simulink model "h"  (R2024a)
settings: Solver=ode45  StartTime=0.0  StopTime=1.5  RelTol=1e-3
PreLoadFcn:
  | power_PVarray_250kW_param;
InitFcn:
  | power_PVarray_250kW_param;
undefined symbols (not defined in the file or in its folder): Clink, D1, Delta, Fc, Fnom, Increment_MPPT, k1, k2, Ki_Ireg, Ki_VDCreg, Kp_Ireg, Kp_VDCreg, LimitL_Ireg, Limits_MPPT, LimitU_Ireg, Pnom, Pnom_xfo, RL, RLff, sigbuilder_block, Ts_Control, Ts_Power, Vf, Vfd, Vnom_dc, Vnom_prim, Vnom_sec
libraries: spsThreePhaseParallelRLCLoadLib x3, spsSeriesRLCBranchLib x3, spsThreePhaseTransformerTwoWindingsLib x2, spsDistributedParametersLineLib x2, eeGeneralControl x2, slpidlib x2, spsabctodq0Lib x2, spsMeanLib x2, spsVoltageMeasurementLib x2, spsThreePhaseSourceLib x1, spsThreeLevelBridgeLib x1, spsThreePhaseVIMeasurementLib x1
Description:
  | Copyright 2008-2018 The MathWorks, Inc.
settings Model: Creator=MathWorks  LastModifiedBy=Ahmed
settings SolverCC: AlgebraicLoopSolver=TrustRegion
settings DataIOCC: LimitDataPoints=on  SaveFormat=Array  SignalLoggingSaveFormat=ModelDataLogs  SignalLogging=off  DSMLogging=off  ReturnWorkspaceOutputs=off
settings OptimizationCC: ExpressionDepthLimit=2147483647  LifeSpan=inf
settings DebuggingCC: UnderspecifiedInitializationDetection=Classic  MergeDetectMultiDrivingBlocksExec=none  SolverPrmCheckMsg=warning  FcnCallInpInsideContextMsg=warning  UnconnectedInputMsg=warning  UnconnectedOutputMsg=warning  UnconnectedLineMsg=warning  StateNameClashWarn=warning  SFUnexpectedBacktrackingDiag=warning  SFNoUnconditionalDefaultTransitionDiag=warning  SFExecutionAtInitializationDiag=none  ArithmeticOperatorsInVariantConditions=warning
settings HardwareCC: ProdBitPerPointer=32  ProdBitPerSizeT=32  ProdBitPerPtrDiffT=32  ProdLargestAtomicFloat=None  ProdIntDivRoundTo=Undefined  ProdEndianess=Unspecified  ProdWordSize=32  ProdHWDeviceType=32-bit Generic
settings ModelReferenceCC: EnableRefExpFcnMdlSchedulingChecks=on  PropagateSignalLabelsOutOfModel=off
settings SFSimCC: SimUseLocalCustomCode=off  CustomCodeUndefinedFunction=UseInterfaceOnly
settings RTWCC: RTWUseLocalCustomCode=off  GPUComputeCapability=3.5
settings CodeAppCC: StateflowObjectComments=on
settings GRTTargetCC: TargetLangStandard=C89/C90 (ANSI)  CombineOutputUpdateFcns=off  GRTInterface=on
settings ConfigComp: CovMetricSettings=dw  CovSaveCumulativeToWorkspaceVar=on  CovSaveSingleToWorkspaceVar=on  CovExternalEMLEnable=off  CovSFcnEnable=off
settings SimscapeCC: SimscapeNormalizeSystem=off

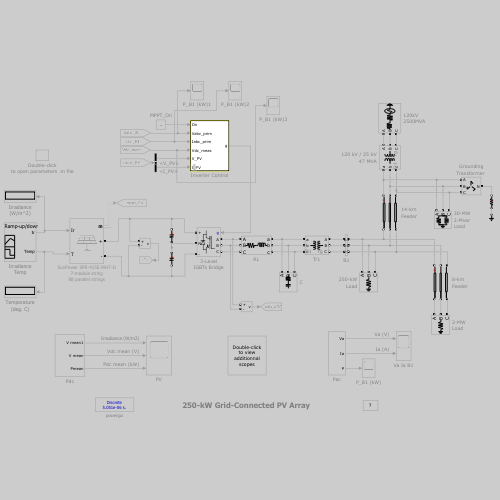
[thumbnail: Simulink's stored preview of the top-level diagram]
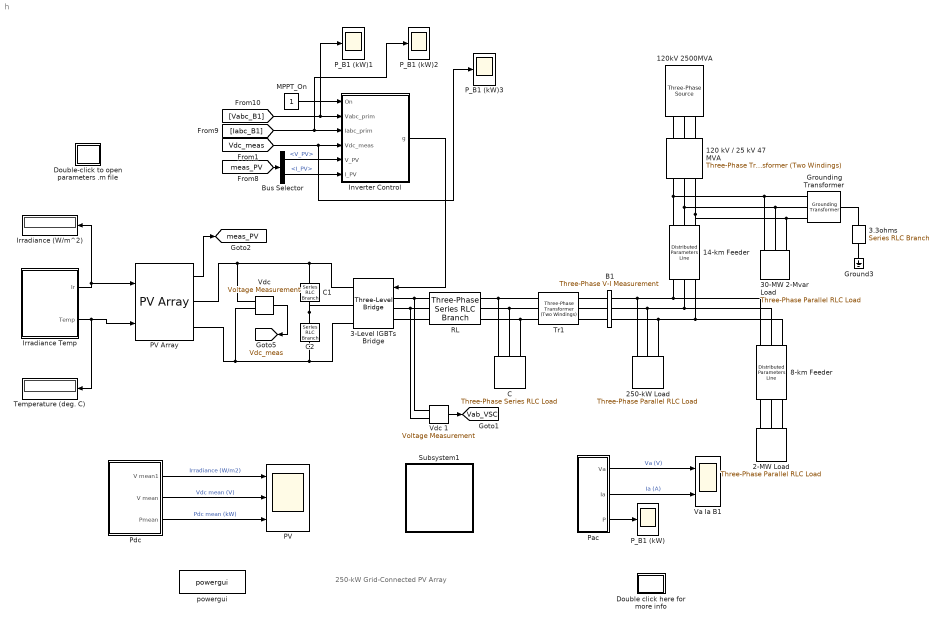
== system h ==
  note: 250-kW Grid-Connected PV Array
  120 kV / 25 kV 47 MVA : spsThreePhaseTransformerTwoWindingsLib/Three-Phase Transformer (Two Windings)  Winding1Connection=Yg  Winding2Connection=Delta (D1)  CoreType=Three single-phase transformers  SetSaturation=off  Hysteresis=off  DataFile='basic_model'  SetInitialFlux=off  Measurements=None  UNITS=pu  NominalPower=[47e6 Fnom ]  Winding1="[ 120e3  0.08/30   0.08 ]"  Winding2="[ Vnom_prim  0.08/30  0.08]"  Rm=500  Lm=500  L0=0.5  Saturation="[ 0,0  ;  0.005,1.2  ;  1.0,1.4 ]"  InitialFluxes=[ 0.8 , -0.8 , 0.7 ]  BreakLoop=off  DiscreteSolver=Trapezoidal iterative  DataType=off  TransfoNumber=0
  120kV 2500MVA : spsThreePhaseSourceLib/Three-Phase Source  InternalConnection=Yg  VoltagePhases=off  Voltage=120e3*1.02  PhaseAngle=0  Voltage_phases=[25e3 25e3 25e3]/sqrt(3)  PhaseAngles_phases=[0 -120 +120]  Frequency=Fnom  NonIdealSource=on  SpecifyImpedance=on  Resistance=0.8929  Inductance=16.58e-3  ShortCircuitLevel=2500e6  BaseVoltage=120e3  XRratio=7  BusType=swing  Pref=0  Qref=0  Prefabc=[10e3, 10e3, 10e3]  Qrefabc=[0, 0, 0]  Qmin=-inf  Qmax=inf
  14-km Feeder : spsDistributedParametersLineLib/Distributed Parameters Line  Phases=3  Length=14  Frequency=Fnom  Resistance=[0.1153 0.413]  Inductance=[1.05e-3 3.32e-3]  Capacitance=[11.33e-009 5.01e-009]  x1=[-6.06060606060606e-05 1.66755797889894e-09 -3576.42610890847 -24705.9443102024;-5.55555555555556e-05 1.66793236560561e-09 -3529.3796467371 -24712.7090235066;-5.05050505050505e-05 1.66830070572728e-09 -3482.32038986587 -24719.3841483486;-4.54545454545455e-05 1.66866299792865e-09 -3435.24850889391 -24725.96966053;-4.04040404040404e-05 1.66901924089635e-09 -3388.16417446609 -24732.4655361767;-3.53535353535354e-05 1.66936943333891e-09 -3341.06755727244 -24738.8717517402;-3.03030303030303e-05 1.66971357398683e-09 -3293.95882804754 -24745.1882839964;-2.52525252525253e-05 1.67005166159252e-09 -3246.83815756985 -24751.4151100468;-2.02020202020202e-05 1.67038369493035e-09 -3199.70571666112 -24757.5522073179;-1.51515151515152e-05 1.67070967279663e-09 -3152.56167618579 -24763.5995535615;-1.01010101010101e-05 1.67102959400963e-09 -3105.40620705033 -24769.5571268547;-5.05050505050505e-06 1.67134345740958e-09 -3058.23948020265 -24775.4249056002]  x2=[-6.06060606060606e-05 1.48154483389501e-09 -4045.01586006552 -24492.383894193;-5.55555555555556e-05 1.48195520050319e-09 -3998.37516636441 -24500.0411868574;-5.05050505050505e-05 1.48236019473042e-09 -3951.71997776183 -24507.6096620227;-4.54545454545455e-05 1.48275981510851e-09 -3905.05046339209 -24515.0892922516;-4.04040404040404e-05 1.48315406018876e-09 -3858.36679244142 -24522.4800504291;-3.53535353535354e-05 1.48354292854195e-09 -3811.66913414736 -24529.7819097622;-3.03030303030303e-05 1.48392641875835e-09 -3764.95765779817 -24536.9948437802;-2.52525252525253e-05 1.48430452944774e-09 -3718.23253273219 -24544.1188263348;-2.02020202020202e-05 1.4846772592394e-09 -3671.49392833726 -24551.1538316001;-1.51515151515152e-05 1.4850446067821e-09 -3624.74201405006 -24558.0998340729;-1.01010101010101e-05 1.48540657074413e-09 -3577.97695935554 -24564.9568085725;-5.05050505050505e-06 1.48576314981331e-09 -3531.19893378629 -24571.724730241]  x3=[-6.06060606060606e-05 -2.31217982093058e-12 0.349732307298334 7.33339900960045;-5.55555555555556e-05 -2.32797013844781e-12 0.335768922746931 7.33405160544255;-5.05050505050505e-05 -2.34375201661246e-12 0.321804320966718 7.3346776138958;-4.54545454545455e-05 -2.35952539821211e-12 0.30783855258214 7.33527703269079;-4.04040404040404e-05 -2.37529022606512e-12 0.293871668221871 7.33584985965453;-3.53535353535354e-05 -2.39104644302087e-12 0.279903718518634 7.33639609271039;-3.03030303030303e-05 -2.40679399195996e-12 0.26593475410901 7.33691572987817;-2.52525252525253e-05 -2.4225328157944e-12 0.251964825633261 7.33740876927409;-2.02020202020202e-05 -2.43826285746784e-12 0.237993983735142 7.33787520911078;-1.51515151515152e-05 -2.45398405995577e-12 0.224022279061721 7.33831504769729;-1.01010101010101e-05 -2.46969636626571e-12 0.210049762263193 7.33872828343915;-5.05050505050505e-06 -2.48539971943746e-12 0.196076483992698 7.33911491483827]  x4=[-6.06060606060606e-05 6.18931442292773e-12 -26.7530894115091 -168.075719805457;-5.55555555555556e-05 6.20822122254007e-12 -26.4330256900655 -168.126352883927;-5.05050505050505e-05 6.22710551612157e-12 -26.1128661436714 -168.176376471088;-4.54545454545455e-05 6.24596723521291e-12 -25.7926119329684 -168.225790385594;-4.04040404040404e-05 6.26480631143663e-12 -25.4722642189416 -168.274594448309;-3.53535353535354e-05 6.28362267649735e-12 -25.1518241629147 -168.32278848231;-3.03030303030303e-05 6.30241626218203e-12 -24.8312929265464 -168.370372312882;-2.52525252525253e-05 6.32118700036019e-12 -24.5106716718259 -168.417345767526;-2.02020202020202e-05 6.33993482298419e-12 -24.1899615610687 -168.463708675954;-1.51515151515152e-05 6.35865966208947e-12 -23.8691637569124 -168.50946087009;-1.01010101010101e-05 6.37736144979478e-12 -23.5482794223126 -168.554602184074;-5.05050505050505e-06 6.39604011830243e-12 -23.2273097205385 -168.599132454259]  x5=5.70973484498186e-05  V1=ones(3,3)  V2=ones(3,3)  I1=ones(3,3)  I2=ones(3,3)  nHarmo=1  Measurements=None  Decoupling=off  VsMag0=0  VrMag0=0  VsAngle0=0  VrAngle0=0  IsMag0=0  IrMag0=0  IsAngle0=0  IrAngle0=0
      settings: LibrarySourceBlock=sps_lib/Power Grid Elements/Distributed Parameters Line
  2-MW Load : spsThreePhaseParallelRLCLoadLib/Three-Phase Parallel RLC Load  LConnTagsString=A|B|C  Configuration=Y (grounded)  NominalVoltage=Vnom_prim  Vabc=[1e3 1e3 1e3]  Vabcp=[1e3 1e3 1e3]  NominalFrequency=Fnom  UnbalancedPower=off  ActivePower=2e6  InductivePower=0  CapacitivePower=0  Pabc=[10e3 9e3 11e3]  QLabc=[100 90 110]  QCabc=[100 90 110]  Pabcp=[10e3 9e3 11e3]  QLabcp=[100 90 110]  QCabcp=[100 90 110]  Measurements=None  LoadType=constant Z
  250-kW Load : spsThreePhaseParallelRLCLoadLib/Three-Phase Parallel RLC Load  LConnTagsString=A|B|C  Configuration=Y (grounded)  NominalVoltage=Vnom_prim  Vabc=[1e3 1e3 1e3]  Vabcp=[1e3 1e3 1e3]  NominalFrequency=Fnom  UnbalancedPower=off  ActivePower=250e3  InductivePower=0  CapacitivePower=0  Pabc=[10e3 9e3 11e3]  QLabc=[100 90 110]  QCabc=[100 90 110]  Pabcp=[10e3 9e3 11e3]  QLabcp=[100 90 110]  QCabcp=[100 90 110]  Measurements=None  LoadType=constant Z
  3-Level IGBTs Bridge : spsThreeLevelBridgeLib/Three-Level Bridge  Arms=3  SnubberResistance=Rs  SbubberCapacitance=Cs  Device=IGBT / Diodes  Ron=Ron  ForwardVoltages="[  Vfd  Vf ]"  Measurements=None
      settings: AttributesFormatString=\n  LibrarySourceBlock=sps_lib/Power Electronics/Three-Level Bridge
  "3.3ohms " : spsSeriesRLCBranchLib/Series RLC Branch  LConnTagsString=__new0  RConnTagsString=__new0  BranchType=R  Resistance=3.3  Inductance=[]  SetiL0=off  InitialCurrent=0  Capacitance=[]  Setx0=off  InitialVoltage=0  Measurements=None
  30-MW 2-Mvar Load : spsThreePhaseParallelRLCLoadLib/Three-Phase Parallel RLC Load  LConnTagsString=A|B|C  Configuration=Y (grounded)  NominalVoltage=Vnom_prim  Vabc=[1e3 1e3 1e3]  Vabcp=[1e3 1e3 1e3]  NominalFrequency=Fnom  UnbalancedPower=off  ActivePower=30e6  InductivePower=2e6  CapacitivePower=0  Pabc=[10e3 9e3 11e3]  QLabc=[100 90 110]  QCabc=[100 90 110]  Pabcp=[10e3 9e3 11e3]  QLabcp=[100 90 110]  QCabcp=[100 90 110]  Measurements=None  LoadType=constant Z
  8-km Feeder : spsDistributedParametersLineLib/Distributed Parameters Line  Phases=3  Length=8  Frequency=Fnom  Resistance=[0.1153 0.413]  Inductance=[1.05e-3 3.32e-3]  Capacitance=[11.33e-009 5.01e-009]  x1=[-3.53535353535354e-05 1.48353383752332e-09 -3811.66913414736 -24529.7819097622;-3.03030303030303e-05 1.48391862639546e-09 -3764.95765779817 -24536.9948437802;-2.52525252525253e-05 1.48429803576885e-09 -3718.23253273219 -24544.1188263348;-2.02020202020202e-05 1.48467206426803e-09 -3671.49392833726 -24551.1538316001;-1.51515151515152e-05 1.48504071053709e-09 -3624.74201405006 -24558.0998340729;-1.01010101010101e-05 1.48540397323962e-09 -3577.97695935554 -24564.9568085725;-5.05050505050505e-06 1.4857618510587e-09 -3531.19893378629 -24571.724730241]  x2=[-3.53535353535354e-05 1.47375181120685e-09 -4047.76151412026 -24417.9507638791;-3.03030303030303e-05 1.47423465072407e-09 -4001.26253570546 -24425.6134191708;-2.52525252525253e-05 1.47471214584885e-09 -3954.74905192191 -24433.1875267788;-2.02020202020202e-05 1.47518429485019e-09 -3908.22123139021 -24440.6730592455;-1.51515151515152e-05 1.47565109601645e-09 -3861.67924278292 -24448.0699894343;-1.01010101010101e-05 1.47611254765538e-09 -3815.12325482394 -24455.3782905298;-5.05050505050505e-06 1.47656864809413e-09 -3768.55343628797 -24462.5979360382]  x3=[-3.53535353535354e-05 -2.50989912594282e-12 -0.394277356463755 -2.24142141422419;-3.03030303030303e-05 -2.50696510265569e-12 -0.390008987982499 -2.2421680533037;-2.52525252525253e-05 -2.5040219911238e-12 -0.385739205641458 -2.24290656408017;-2.02020202020202e-05 -2.50106980201652e-12 -0.381468024919441 -2.24363694387637;-1.51515151515152e-05 -2.49810854603612e-12 -0.377195461300321 -2.24435919004451;-1.01010101010101e-05 -2.49513823391774e-12 -0.372921530272988 -2.24507329996632;-5.05050505050505e-06 -2.49215887642935e-12 -0.368646247331288 -2.24577927105301]  x4=[-3.53535353535354e-05 6.37625008259566e-12 -26.1994856823162 -158.047293349204;-3.03030303030303e-05 6.3771294739055e-12 -25.89851703212 -158.096890546791;-2.52525252525253e-05 6.37798574685863e-12 -25.5974544946729 -158.145914611856;-2.02020202020202e-05 6.37881889835091e-12 -25.2962991613863 -158.194365366674;-1.51515151515152e-05 6.379628925362e-12 -24.9950521240077 -158.242242635604;-1.01010101010101e-05 6.38041582495538e-12 -24.6937144746175 -158.28954624508;-5.05050505050505e-06 6.38117959427839e-12 -24.3922873056242 -158.336276023617]  x5=3.26270562570392e-05  V1=ones(3,3)  V2=ones(3,3)  I1=ones(3,3)  I2=ones(3,3)  nHarmo=1  Measurements=None  Decoupling=off  VsMag0=0  VrMag0=0  VsAngle0=0  VrAngle0=0  IsMag0=0  IrMag0=0  IsAngle0=0  IrAngle0=0
      settings: LibrarySourceBlock=sps_lib/Power Grid Elements/Distributed Parameters Line
  B1 : spsThreePhaseVIMeasurementLib/Three-Phase V-I Measurement  VoltageMeasurement=phase-to-ground  SetLabelV=on  LabelV=Vabc_B1  Vpu=off  VpuLL=off  CurrentMeasurement=yes  SetLabelI=on  LabelI=Iabc_B1  Ipu=off  Pbase=100e6  Vbase=500e3  OutputType=Magnitude  PhasorSimulation=off  PSBequivalent=0
  Bus Selector : BusSelector  OutputSignals=V_PV,I_PV
  C : spsThreePhaseSeriesRLCLoadLib/Three-Phase Series RLC Load  LConnTagsString=A|B|C  Configuration=Delta  NominalVoltage=Vnom_sec  Vabc=[1e3 1e3 1e3]  Vabcp=[1e3 1e3 1e3]  NominalFrequency=Fnom  UnbalancedPower=off  ActivePower=Pc  InductivePower=0  CapacitivePower=Qc  Pabc=[10e3 9e3 11e3]  QLabc=[100 90 110]  QCabc=[100 90 110]  Pabcp=[10e3 9e3 11e3]  QLabcp=[100 90 110]  QCabcp=[100 90 110]  Measurements=None  LoadType=constant Z
  C1 : spsSeriesRLCBranchLib/Series RLC Branch  LConnTagsString=__new0  RConnTagsString=__new0  BranchType=C  Resistance=1.0  Inductance=1.0  SetiL0=off  InitialCurrent=0  Capacitance=Clink  Setx0=on  InitialVoltage=Vnom_dc/2  Measurements=None
  C2 : spsSeriesRLCBranchLib/Series RLC Branch  LConnTagsString=__new0  RConnTagsString=__new0  BranchType=C  Resistance=1.0  Inductance=1.0  SetiL0=off  InitialCurrent=0  Capacitance=Clink  Setx0=on  InitialVoltage=Vnom_dc/2  Measurements=None
  Double click here for more info : Subsystem
      settings: OpenFcn=showdemo(bdroot(gcb))
      mask Display: disp('?')
  Double-click to open parameters .m file : Subsystem
      settings: OpenFcn=open('power_PVarray_250kW_param.m')
  Ground3 : spsGroundLib/Ground  LConnTagsString=a
  "Grounding Transformer " : spsGroundingTransformerLib/Grounding Transformer   UNITS=pu  NominalPower="[100e6   Fnom]"  NominalVoltage=Vnom_prim  ZeroSequenceImpedance_pu=[0.025 0.75]  MagnetizationBranch_pu=[500 500]  ZeroSequenceImpedance_SI=[0.052083 589.05]  MagnetizationBranch_SI=[1041.7 3.927e+005]  Measurements=None
      settings: LibrarySourceBlock=|
      | sps_lib/Power Grid Elements/Grounding
      | Transformer
  Inverter Control : Subsystem  mask(Inverter Control){Pnom=Pnom, Fnom=Fnom, Vnom_prim=Vnom_prim, Vnom_sec=Vnom_sec, Vnom_dc=Vnom_dc, Increment_MPPT=Increment_MPPT, Limits_MPPT=Limits_MPPT, Vdc_ref_Init=Vnom_dc, Kp_VDCreg=Kp_VDCreg, Ki_VDCreg=Ki_VDCreg, Kp_Ireg=Kp_Ireg, Ki_Ireg=Ki_Ireg, RLff=RLff, Fc=Fc, Ts_Control=Ts_Control, Ts_PWMgenerator=Ts_Power}
      mask prompts: Pnom "Power (VA)"; Fnom "Frequency (Hz)"; Vnom_prim "Primary voltage (Vrms LL)"; Vnom_sec "Secondary voltage (Vrms LL)"; Vnom_dc "DC voltage (V)"; Increment_MPPT "Output increment (V)"; Limits_MPPT "Output limits [ Upper  Lower ]"; Vdc_ref_Init "Output initial value (V)"; Kp_VDCreg "Proportional gain"; Ki_VDCreg "Integral gain"; Kp_Ireg "Proportional gain"; Ki_Ireg "Integral gain"; RLff "Feedforward Values [Rff Lff]"; Fc "Carrier frequency (Hz)"; Ts_Control "Control systems"; Ts_PWMgenerator "PWM generator"
      mask help:
      | The main components of the Inverter Control are:
      | 1. PLL & Measurements
      | 2. Maximum Power Point Tracker System (MPPT) using a Perturb & Observe algorithm
      | 3. DC Voltage Regulator
      | 4. Current Regulator
      | 5. PWM Modulator
      mask DialogControl Container4 Prompt: Nominal Values:
      mask DialogControl Container3 Prompt: MPPT Controller:
      mask DialogControl Container8 Prompt: Dc Voltage Regulator:
      mask DialogControl Container6 Prompt: Current Regulator:
      mask DialogControl Container9 Prompt: PWM Modulator:
      mask DialogControl SampleTimes Prompt: Sample Times:
  Irradiance (W/m^2) : Display
      settings: Format=bank  Decimation=1000
  Irradiance Temp : Subsystem  Tag=STV Subsys  LoadFcn=sigbuilder_block('load');  StartFcn=sigbuilder_block('start');  StopFcn=sigbuilder_block('stop');  ClipboardFcn=sigbuilder_block('clipboard');  mask(Sigbuilder block){tuvar=[0:10]}
      mask help: Sigbuilder GUI
      mask init:
      | if ~strcmp(get_param(bdroot(gcbh),'SimulationStatus'),'stopped') tuvar = sigbuilder_block('maskInit'); end
      settings: CopyFcn=sigbuilder_block('copy');  DeleteFcn=sigbuilder_block('delete');  ModelCloseFcn=sigbuilder_block('modelClose');  PreSaveFcn=sigbuilder_block('preSave');  PauseFcn=sigbuilder_block('pause')  ContinueFcn=sigbuilder_block('continue')  NameChangeFcn=sigbuilder_block('namechange');  OpenFcn=sigbuilder_block('open',[6 30 756 447.75 ]);  CloseFcn=sigbuilder_block('close');
      mask Display: plot(0, 0, 100, 100,[2, 2, 32, 32, 2], [68, 8, 8, 68, 68],[32, 2], [38, 38], [32, 19, 2],[53, 60, 44], [32, 17, 17, 2],[16, 16, 31, 31]);txt = getActiveGroup(gcbh);text(2, 100, txt,'verticalAlignment', 'top');
  MPPT_On : Constant
  PV : Scope  NumInputPorts=3
  PV Array : spsPVArrayLib/PV Array  Npar=88  Nser=7  PlotType=array @ 1000 W/m2 & specified temperatures  S_vec="[ 1000  500  100 ]"  Temp_C_vec="[ 45 25  ]"  ModuleName=SunPower SPR-415E-WHT-D  PlotWhenSelected=off  Pm=414.801  Ncell=128  Voc=85.3  Isc=6.09  Vm=72.9  Im=5.69  beta_Voc_pc=-0.229  alpha_Isc_pc=0.030706  beta_Voc=-0.19534  alpha_Isc=0.00187  IL=6.0978  I0=7.1698e-13  nI=0.87223  Rsh=419.7781  Rs=0.53711  RobustModel=off  RobustCellTemperature=313.3991  BAL=on  Tc=1e-6  Tfilter=5e-5
      settings: AttributesFormatString=|
      | %<ModuleName>
      | %<Nser>-module string
      | %<Npar> parallel strings
  P_B1 (kW){,1..3} (4 alike) : Scope
  Pac : Subsystem
  Pdc : Subsystem
  RL : spsThreePhaseSeriesRLCBranchLib/Three-Phase Series RLC Branch  LConnTagsString=A|B|C  RConnTagsString=A|B|C  BranchType=RL  Resistance=RL(1)  Inductance=RL(2)  Capacitance=inf  Measurements=None
  Subsystem1 : Subsystem
      mask Display: disp('Double-click\nto view\nadditionnal\nscopes')
  Temperature (deg. C) : Display
      settings: Format=bank  Decimation=1000
  Tr1 : spsThreePhaseTransformerTwoWindingsLib/Three-Phase Transformer (Two Windings)  Winding1Connection=Yg  Winding2Connection=Delta (D1)  CoreType=Three single-phase transformers  SetSaturation=off  Hysteresis=off  DataFile='hysteresis'  SetInitialFlux=off  Measurements=None  UNITS=pu  NominalPower=[Pnom_xfo, Fnom ]  Winding1=W1_xfo  Winding2=W2_xfo  Rm=Rm_xfo  Lm=Lm_xfo  L0=0.5  Saturation=[ 0,0 ; 0.0024,1.2 ; 1.0,1.52 ]  InitialFluxes=[ 0.8 , -0.8 , 0.7 ]  BreakLoop=off  DiscreteSolver=Trapezoidal iterative  DataType=off  TransfoNumber=0
  Va Ia B1 : Scope  NumInputPorts=2
  "Vdc " : spsVoltageMeasurementLib/Voltage Measurement  Tag=PoWeRsYsTeMmEaSuReMeNt  PhasorSimulation=off  OutputType=Magnitude  PSBequivalent=0
  Vdc 1 : spsVoltageMeasurementLib/Voltage Measurement  Tag=PoWeRsYsTeMmEaSuReMeNt  PhasorSimulation=off  OutputType=Magnitude  PSBequivalent=0
  powergui : spspowerguiLib/powergui  Priority=1  SimulationMode=Discrete  SampleTime=Ts_Power  frequency=60  Iterations=50  frequencyindice=0  Pbase=100e6  ErrMax=1e-4  UnitsV=kV  UnitsW=MW  buscounter=0  FunctionMessages=off  echomessages=off  EnableUseOfTLC=off  CurrentSourceSwitches=off  DisableSnubberDevices=off  DisableRonSwitches=off  DisableVfSwitches=off  DisplayEquations=off  AutomaticDiscreteSolvers=off  SolverType=Tustin  Interpol=off  ExternalGateDelay=off  methode=off  Ts=0  x0status=blocks  SPID=off  SwTol=0  HookPort=off  NonlinearTolerance=1e-4  nMaxIteration=100  ContinueOnMaxIteration=off  RestoreLinks=warning  ResistiveCurrentMeasurement=off  Frange=[0:2:500]  Ylog=off  Xlog=on  ShowGrid=off  save=off  variable=ZData  structure=VaIa_Grid  ZoomFFT=off  StartTime=1.4  cycles=3  DisplayStyle=1  fundamental=60  FreqAxis=on  MaxFrequency=5000  frequencyindicesteady=1  RmsSteady=1  display=off
  tag scope: Vab_VSC=global, Vdc_meas=global, meas_PV=global
  wires:
  Vdc 1/1 -> [Vab_VSC]
  Pac/2(Ia) -> Va Ia B1/2  "Ia (A)"
  Pac/1(Va) -> Va Ia B1/1  "Va (V)"
  PV Array/1 -> [meas_PV]
  Inverter Control/1(g) -> 3-Level IGBTs Bridge/1
  [Vabc_B1] -> P_B1 (kW)1/1, Inverter Control/2(Vabc_prim)
  [Iabc_B1] -> P_B1 (kW)2/1, Inverter Control/3(Iabc_prim)
  [Vdc_meas] -> P_B1 (kW)3/1, Inverter Control/4(Vdc_meas)
  [meas_PV] -> Bus Selector/1
  "Vdc "/1 -> [Vdc_meas]
  Bus Selector/1 -> Inverter Control/5(V_PV)  "<V_PV>"
  Bus Selector/2 -> Inverter Control/6(I_PV)  "<I_PV>"
  Pac/3(P) -> P_B1 (kW)/1
  MPPT_On/1 -> Inverter Control/1(On)
  Pdc/2(V mean) -> PV/2  "Vdc mean (V)"
  Pdc/3(Pmean) -> PV/3  "Pdc mean (kW)"
  Pdc/1(V mean1) -> PV/1  "Irradiance (W/m2)"
  Irradiance Temp/1(Ir) -> PV Array/1, Irradiance (W/m^2)/1
  Irradiance Temp/2(Temp) -> PV Array/2, Temperature (deg. C)/1
  connections:
  B1/LConn1 -- Tr1/LConn1
  B1/LConn2 -- Tr1/LConn2
  B1/LConn3 -- Tr1/LConn3
  C2/LConn1 -- 3-Level IGBTs Bridge/RConn2 -- C1/RConn1
  C1/LConn1 -- PV Array/RConn1 -- "Vdc "/LConn1 -- 3-Level IGBTs Bridge/RConn1
  C2/RConn1 -- PV Array/RConn2 -- "Vdc "/LConn2 -- 3-Level IGBTs Bridge/RConn3
  RL/LConn1 -- Vdc 1/LConn1 -- 3-Level IGBTs Bridge/LConn1
  RL/LConn2 -- Vdc 1/LConn2 -- 3-Level IGBTs Bridge/LConn2
  RL/LConn3 -- 3-Level IGBTs Bridge/LConn3
  RL/RConn1 -- Tr1/RConn1 -- C/LConn1
  RL/RConn2 -- Tr1/RConn2 -- C/LConn2
  RL/RConn3 -- Tr1/RConn3 -- C/LConn3
  "Grounding Transformer "/RConn1 -- "3.3ohms "/LConn1
  "3.3ohms "/RConn1 -- Ground3/LConn1
  120 kV / 25 kV 47 MVA/RConn1 -- 14-km Feeder/LConn1 -- 30-MW 2-Mvar Load/LConn1 -- "Grounding Transformer "/LConn1
  120 kV / 25 kV 47 MVA/RConn2 -- 30-MW 2-Mvar Load/LConn2 -- "Grounding Transformer "/LConn2 -- 14-km Feeder/LConn2
  120 kV / 25 kV 47 MVA/RConn3 -- 30-MW 2-Mvar Load/LConn3 -- "Grounding Transformer "/LConn3 -- 14-km Feeder/LConn3
  120kV 2500MVA/RConn1 -- 120 kV / 25 kV 47 MVA/LConn1
  120kV 2500MVA/RConn2 -- 120 kV / 25 kV 47 MVA/LConn2
  120kV 2500MVA/RConn3 -- 120 kV / 25 kV 47 MVA/LConn3
  14-km Feeder/RConn1 -- B1/RConn1 -- 250-kW Load/LConn1 -- 8-km Feeder/LConn1
  14-km Feeder/RConn2 -- B1/RConn2 -- 250-kW Load/LConn2 -- 8-km Feeder/LConn2
  14-km Feeder/RConn3 -- B1/RConn3 -- 250-kW Load/LConn3 -- 8-km Feeder/LConn3
  2-MW Load/LConn1 -- 8-km Feeder/RConn1
  2-MW Load/LConn2 -- 8-km Feeder/RConn2
  2-MW Load/LConn3 -- 8-km Feeder/RConn3

== system h/Double click here for more info ==

== system h/Double-click to open parameters .m file ==

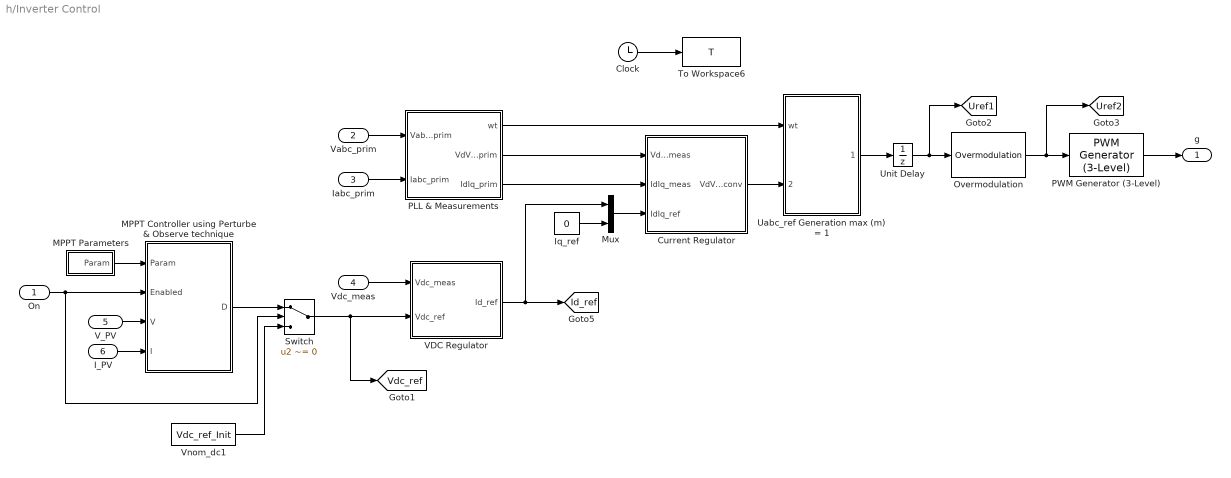
== system h/Inverter Control ==
  On : Inport  PortDimensions=1
  Vabc_prim : Inport  Port=2  PortDimensions=3
  Iabc_prim : Inport  Port=3  PortDimensions=3
  Vdc_meas : Inport  Port=4  PortDimensions=1
  V_PV : Inport  Port=5  PortDimensions=1
  I_PV : Inport  Port=6  PortDimensions=1
  Clock : Clock
      settings: Decimation=30
  Current Regulator : Subsystem
  Iq_ref : Constant  Value=0
  MPPT Parameters : Subsystem
  "MPPT Controller using Perturbe & Observe technique " : MATLAB Function  TreatAsAtomicUnit=on
  Mux : Mux  Inputs=2
  Overmodulation : spsOvermodulationLib/Overmodulation  OverModType=Flat top
      settings: LibrarySourceBlock=sps_lib/Power Electronics/Power Electronics Control/Overmodulation
  PLL & Measurements : Subsystem
  PWM Generator (3-Level) : spsPWMGenerator3LevelLib/PWM Generator (3-Level)  ModulatorType=Three-phase bridge (12 pulses)  ModulatorMode=Unsynchronized  nF=27  Fc=Fc  ModulatingSignals=off  m=0.8  Freq=60  Phase=0  Ts=Ts_PWMgenerator
      settings: LibrarySourceBlock=|
      | sps_lib/Power Electronics/Power Electronics Control/PWM Generator
      | (3-Level)
  Switch : Switch  Criteria=u2 ~= 0  SaturateOnIntegerOverflow=off  InputSameDT=off
  To Workspace6 : ToWorkspace  VariableName=T  SampleTime=-1
  Uabc_ref Generation max (m) = 1 : Subsystem
  Unit Delay : UnitDelay  SampleTime=Ts_Control  HasFrameUpgradeWarning=on
  VDC Regulator : Subsystem
  Vnom_dc1 : Constant  Value=Vdc_ref_Init
  g : Outport  VectorParamsAs1DForOutWhenUnconnected=off
  tag scope: Id_ref=global, Uref1=global, Uref2=global, Vdc_ref=global
  wires:
  PLL & Measurements/1(wt) -> Uabc_ref Generation max (m) = 1/1(wt)
  Current Regulator/1(VdVq_conv) -> Uabc_ref Generation max (m) = 1/2(VdVq_conv)
  Iq_ref/1 -> Mux/2
  Mux/1 -> Current Regulator/3(IdIq_ref)
  PLL & Measurements/3(IdIq_prim) -> Current Regulator/2(IdIq_meas)
  PLL & Measurements/2(VdVq_prim) -> Current Regulator/1(VdVq_meas)
  Vabc_prim/1 -> PLL & Measurements/1(Vabc_prim)
  Iabc_prim/1 -> PLL & Measurements/2(Iabc_prim)
  PWM Generator (3-Level)/1 -> g/1
  Vdc_meas/1 -> VDC Regulator/1(Vdc_meas)
  VDC Regulator/1(Id_ref) -> [Id_ref], Mux/1
  V_PV/1 -> "MPPT Controller using Perturbe & Observe technique "/3(V)
  I_PV/1 -> "MPPT Controller using Perturbe & Observe technique "/4(I)
  MPPT Parameters/1(Param) -> "MPPT Controller using Perturbe & Observe technique "/1(Param)
  On/1 -> "MPPT Controller using Perturbe & Observe technique "/2(Enabled), Switch/2
  Overmodulation/1 -> [Uref2], PWM Generator (3-Level)/1
  Unit Delay/1 -> [Uref1], Overmodulation/1
  "MPPT Controller using Perturbe & Observe technique "/1(D) -> Switch/1
  Switch/1 -> [Vdc_ref], VDC Regulator/2(Vdc_ref)
  Vnom_dc1/1 -> Switch/3
  Uabc_ref Generation max (m) = 1/1(Uabc_ref) -> Unit Delay/1
  Clock/1 -> To Workspace6/1

== system h/Irradiance Temp ==
  Demux : Demux  Tag=STV Demux  Outputs=2
      settings: DisplayOption=none
  FromWs : FromWorkspace  Tag=STV FromWs  VariableName=tuvar
      SigBuilderData=|
      | common.afterFinalStr = 'Extrapolate'
      | common.sampleTime = '0'
      | dataSet(1).timeRange = [0 2]
      | dataSet(1).name = 'Constant Irradiance'
      | dataSet(2).timeRange = [0 2]
      | dataSet(2).name = 'Step Irradiance'
      | dataSet(3).timeRange = [0 6.5]
      | dataSet(3).name = 'Ramp-up/down Irradiance'
      | sbobj.Groups(1).Name = 'Constant Irradiance'
      | sbobj.Groups(1).Signals(1).Name = 'Ir'
      | sbobj.Groups(1).Signals(1).XData = [0 2]
      | sbobj.Groups(1).Signals(1).YData = [1000 1000]
      | sbobj.Groups(1).Signals(2).Name = 'Temp'
      | sbobj.Groups(1).Signals(2).XData = [0 1 1 2]
      | sbobj.Groups(1).Signals(2).YData = [0 0 1 1]
      | sbobj.Groups(1).TimeRange = [0 2]
      | sbobj.Groups(2).Name = 'Step Irradiance'
      | sbobj.Groups(2).Signals(1).Name = 'Ir'
      | sbobj.Groups(2).Signals(1).XData = [0 0.252 0.252 2]
      | sbobj.Groups(2).Signals(1).YData = [600 600 1000 1000]
      | sbobj.Groups(2).Signals(2).Name = 'Temp'
      | sbobj.Groups(2).Signals(2).XData = [0 1 1 2]
      | sbobj.Groups(2).Signals(2).YData = [0 0 1 1]
      | sbobj.Groups(2).TimeRange = [0 2]
      | sbobj.Groups(3).Name = 'Ramp-up/down Irradiance'
      | sbobj.Groups(3).Signals(1).Name = 'Ir'
      | sbobj.Groups(3).Signals(1).XData = [0 0.5 0.5 1 1 1.5 1.5 2.5 3 6.5]
      | sbobj.Groups(3).Signals(1).YData = [795 795 1000 995 400 400 120 600 900 900]
      | sbobj.Groups(3).Signals(2).Name = 'Temp'
      | sbobj.Groups(3).Signals(2).XData = [0 0.7 1 6.5]
      | sbobj.Groups(3).Signals(2).YData = [25 25 50 50]
      | sbobj.Groups(3).TimeRange = [0 6.5]
  Ir : Outport  Tag=STV Outport  VectorParamsAs1DForOutWhenUnconnected=off
  Temp : Outport  Tag=STV Outport  Port=2  VectorParamsAs1DForOutWhenUnconnected=off
  wires:
  Demux/1 -> Ir/1
  FromWs/1 -> Demux/1
  Demux/2 -> Temp/1

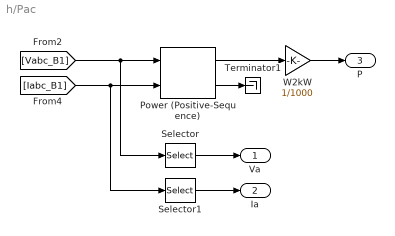
== system h/Pac ==
  Power (Positive-Sequence) : spsPowerPositiveSequenceLib/Power (Positive-Sequence)  Freq=60  Vinit=[0, 0]  Iinit=[0, 0]  Ts=Ts_Control
      settings: LibrarySourceBlock=|
      | sps_lib/Sensors and Measurements/Power
      | (Positive-Sequence)
  Selector : Selector  InputPortWidth=3  IndexOptions=Index vector (dialog)  Indices=[1]  OutputSizes=1
  Selector1 : Selector  InputPortWidth=3  IndexOptions=Index vector (dialog)  Indices=[1]  OutputSizes=1
  Terminator1 : Terminator
  W2kW : Gain  Gain=1/1000
  Va : Outport  VectorParamsAs1DForOutWhenUnconnected=off
  Ia : Outport  Port=2  VectorParamsAs1DForOutWhenUnconnected=off
  P : Outport  Port=3  VectorParamsAs1DForOutWhenUnconnected=off
  wires:
  Power (Positive-Sequence)/2 -> Terminator1/1
  W2kW/1 -> P/1
  Power (Positive-Sequence)/1 -> W2kW/1
  [Iabc_B1] -> Selector1/1, Power (Positive-Sequence)/2
  [Vabc_B1] -> Selector/1, Power (Positive-Sequence)/1
  Selector/1 -> Va/1
  Selector1/1 -> Ia/1

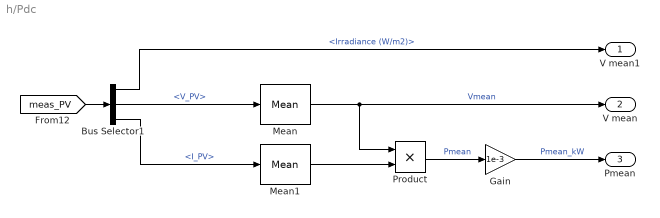
== system h/Pdc ==
  Bus Selector1 : BusSelector  OutputSignals=Irradiance (W/m2),V_PV,I_PV
  Gain : Gain  Gain=1e-3
  Mean : spsMeanLib/Mean  Freq=Fnom  Vinit=Vnom_dc/2  Ts=Ts_Control
  Mean1 : spsMeanLib/Mean  Freq=Fnom  Vinit=0  Ts=Ts_Control
  Product : Product
  V mean1 : Outport  VectorParamsAs1DForOutWhenUnconnected=off
  V mean : Outport  Port=2  VectorParamsAs1DForOutWhenUnconnected=off
  Pmean : Outport  Port=3  VectorParamsAs1DForOutWhenUnconnected=off
  wires:
  Mean/1 -> V mean/1, Product/1  "Vmean"
  Mean1/1 -> Product/2
  Product/1 -> Gain/1  "Pmean"
  Gain/1 -> Pmean/1  "Pmean_kW"
  Bus Selector1/2 -> Mean/1  "<V_PV>"
  Bus Selector1/3 -> Mean1/1  "<I_PV>"
  [meas_PV] -> Bus Selector1/1
  Bus Selector1/1 -> V mean1/1  "<Irradiance (W/m2)>"

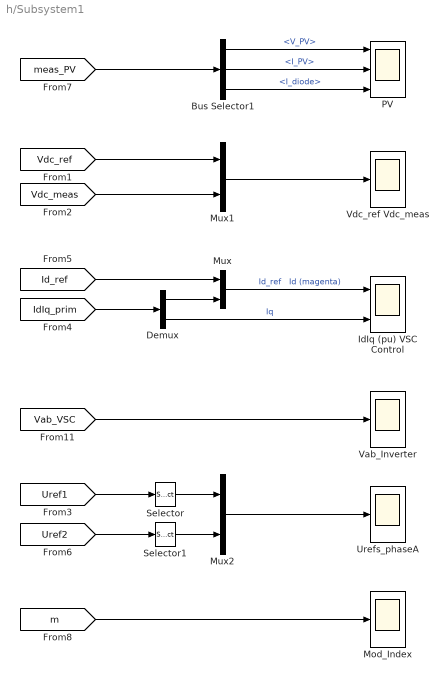
== system h/Subsystem1 ==
  Bus Selector1 : BusSelector  OutputSignals=V_PV,I_PV,I_diode
  Demux : Demux  Outputs=2
  IdIq (pu) VSC Control : Scope  NumInputPorts=2
  Mod_Index : Scope
  Mux : Mux  Inputs=2
  Mux1 : Mux  Inputs=2
  Mux2 : Mux  Inputs=2
  PV : Scope  NumInputPorts=3
  Selector : Selector  InputPortWidth=3  IndexOptions=Index vector (dialog)  Indices=[1]  OutputSizes=1
  Selector1 : Selector  InputPortWidth=3  IndexOptions=Index vector (dialog)  Indices=[1]  OutputSizes=1
  Urefs_phaseA : Scope
  Vab_Inverter : Scope
  Vdc_ref Vdc_meas : Scope
  wires:
  [IdIq_prim] -> Demux/1
  [Id_ref] -> Mux/1
  Demux/1 -> Mux/2
  Mux/1 -> IdIq (pu) VSC Control/1  "Id_ref   Id (magenta)"
  Demux/2 -> IdIq (pu) VSC Control/2  "Iq"
  [Vdc_ref] -> Mux1/1
  [Vdc_meas] -> Mux1/2
  Mux1/1 -> Vdc_ref Vdc_meas/1
  [Vab_VSC] -> Vab_Inverter/1
  [meas_PV] -> Bus Selector1/1
  Bus Selector1/3 -> PV/3  "<I_diode>"
  Bus Selector1/1 -> PV/1  "<V_PV>"
  Bus Selector1/2 -> PV/2  "<I_PV>"
  [Uref1] -> Selector/1
  [Uref2] -> Selector1/1
  Mux2/1 -> Urefs_phaseA/1
  Selector/1 -> Mux2/1
  Selector1/1 -> Mux2/2
  [m] -> Mod_Index/1

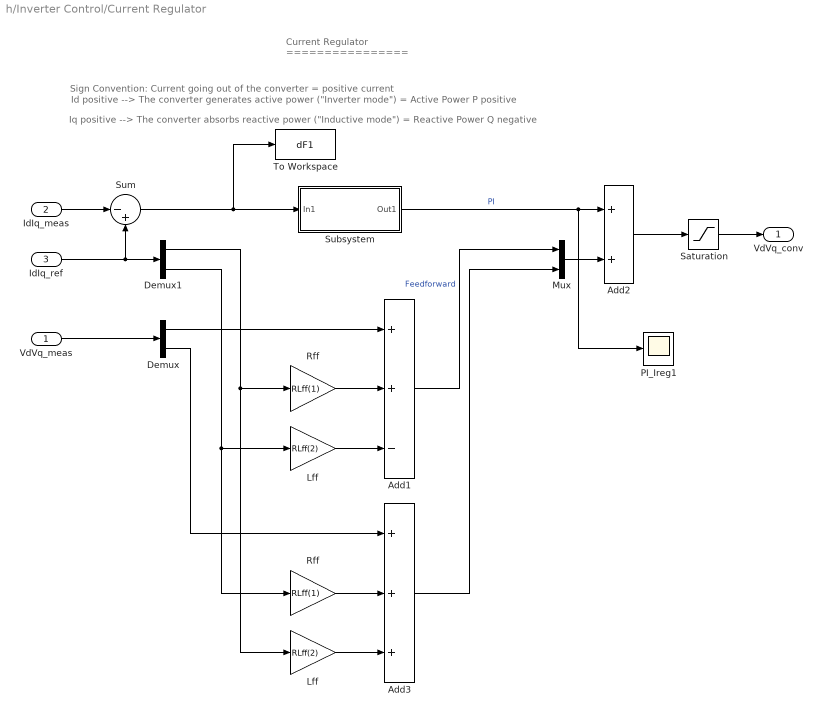
== system h/Inverter Control/Current Regulator ==
  note: Current Regulator
      | ================
  note: Sign Convention: Current going out of the converter = positive current
  note: Iq positive --> The converter absorbs reactive power ("Inductive mode") = Reactive Power Q negative
  note: Id positive --> The converter generates active power ("Inverter mode") = Active Power P positive
  VdVq_meas : Inport  PortDimensions=2
  IdIq_meas : Inport  Port=2  PortDimensions=2
  IdIq_ref : Inport  Port=3  PortDimensions=2
  Add1 : Sum  Inputs=++-
  Add2 : Sum
  Add3 : Sum  Inputs=+++
  Demux : Demux  Outputs=2
  Demux1 : Demux  Outputs=2
  Lff : Gain  Gain=RLff(2)  SaturateOnIntegerOverflow=on  OutDataTypeStr=Inherit: Same as input  ParamDataTypeStr=Inherit: Same as input
  "Lff  " : Gain  Gain=RLff(2)  SaturateOnIntegerOverflow=on  OutDataTypeStr=Inherit: Same as input  ParamDataTypeStr=Inherit: Same as input
  Mux : Mux  Inputs=2
  PI_Ireg1 : Scope
  Rff : Gain  Gain=RLff(1)  SaturateOnIntegerOverflow=on  OutDataTypeStr=Inherit: Same as input  ParamDataTypeStr=Inherit: Same as input
  "Rff " : Gain  Gain=RLff(1)  SaturateOnIntegerOverflow=on  OutDataTypeStr=Inherit: Same as input  ParamDataTypeStr=Inherit: Same as input
  Saturation : Saturate  UpperLimit=LimitU_Ireg  LowerLimit=LimitL_Ireg
  Subsystem : Subsystem
  Sum : Sum  Inputs=|-+
  To Workspace : ToWorkspace  VariableName=dF1  SampleTime=-1
  VdVq_conv : Outport  VectorParamsAs1DForOutWhenUnconnected=off
  wires:
  Mux/1 -> Add2/2
  Subsystem/1(Out1) -> PI_Ireg1/1, Add2/1  "PI"
  IdIq_ref/1 -> Sum/2, Demux1/1
  IdIq_meas/1 -> Sum/1
  Add2/1 -> Saturation/1
  Saturation/1 -> VdVq_conv/1
  VdVq_meas/1 -> Demux/1
  Demux/1 -> Add1/1
  "Rff "/1 -> Add1/2
  Demux1/1 -> "Rff "/1, Lff/1
  "Lff  "/1 -> Add1/3
  Demux1/2 -> "Lff  "/1, Rff/1
  Rff/1 -> Add3/2
  Lff/1 -> Add3/3
  Add1/1 -> Mux/1  "Feedforward"
  Demux/2 -> Add3/1
  Add3/1 -> Mux/2
  Sum/1 -> Subsystem/1(In1), To Workspace/1

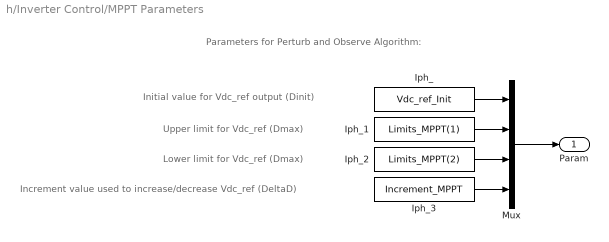
== system h/Inverter Control/MPPT Parameters ==
  note: Parameters for Perturb and Observe Algorithm:
  note: Lower limit for Vdc_ref (Dmax)
  note: Initial value for Vdc_ref output (Dinit)
  note: Increment value used to increase/decrease Vdc_ref (DeltaD)
  note: Upper limit for Vdc_ref (Dmax)
  Iph_ : Constant  Value=Vdc_ref_Init
  Iph_1 : Constant  Value=Limits_MPPT(1)
  Iph_2 : Constant  Value=Limits_MPPT(2)
  Iph_3 : Constant  Value=Increment_MPPT
  Mux : Mux
  Param : Outport  VectorParamsAs1DForOutWhenUnconnected=off
  wires:
  Mux/1 -> Param/1
  Iph_3/1 -> Mux/4
  Iph_2/1 -> Mux/3
  Iph_1/1 -> Mux/2
  Iph_/1 -> Mux/1

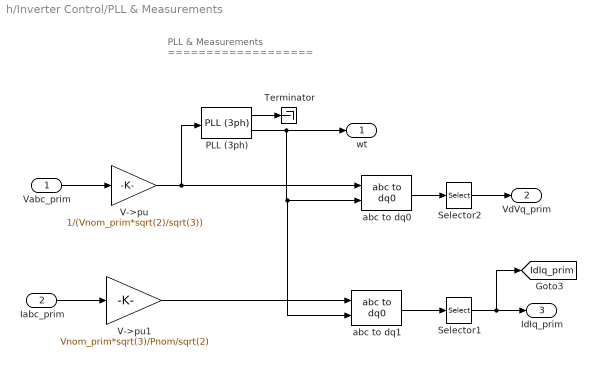
== system h/Inverter Control/PLL & Measurements ==
  note: PLL & Measurements
      | ===================
  Vabc_prim : Inport
  Iabc_prim : Inport  Port=2
  PLL (3ph) : spsPLL3phLib/PLL (3ph)  Fmin=45  Par_Init="[-0.57  Fnom]"  ParK=[180, 3200, 1]  TcD=1e-4  MaxRateChangeFreq=12  FilterCutOffFreq=25  Ts=Ts_Control  AGC=on
  Selector1 : Selector  InputPortWidth=3  IndexOptions=Index vector (dialog)  Indices=[1 2]  OutputSizes=1
  Selector2 : Selector  InputPortWidth=3  IndexOptions=Index vector (dialog)  Indices=[1 2]  OutputSizes=1
  Terminator : Terminator
  V->pu : Gain  Gain=1/(Vnom_prim*sqrt(2)/sqrt(3))  SaturateOnIntegerOverflow=on  OutDataTypeStr=Inherit: Same as input  ParamDataTypeStr=Inherit: Same as input
  V->pu1 : Gain  Gain=Vnom_prim*sqrt(3)/Pnom/sqrt(2)  SaturateOnIntegerOverflow=on  OutDataTypeStr=Inherit: Same as input  ParamDataTypeStr=Inherit: Same as input
  abc to dq0 : spsabctodq0Lib/abc to dq0  Alignment=90 degrees behind phase A axis
  abc to dq1 : spsabctodq0Lib/abc to dq0  Alignment=90 degrees behind phase A axis
  wt : Outport  VectorParamsAs1DForOutWhenUnconnected=off
  VdVq_prim : Outport  Port=2  VectorParamsAs1DForOutWhenUnconnected=off
  IdIq_prim : Outport  Port=3  VectorParamsAs1DForOutWhenUnconnected=off
  tag scope: IdIq_prim=global
  wires:
  V->pu1/1 -> abc to dq1/1
  V->pu/1 -> PLL (3ph)/1, abc to dq0/1
  abc to dq1/1 -> Selector1/1
  Vabc_prim/1 -> V->pu/1
  Iabc_prim/1 -> V->pu1/1
  abc to dq0/1 -> Selector2/1
  Selector2/1 -> VdVq_prim/1
  Selector1/1 -> [IdIq_prim], IdIq_prim/1
  PLL (3ph)/2 -> wt/1, abc to dq1/2, abc to dq0/2
  PLL (3ph)/1 -> Terminator/1

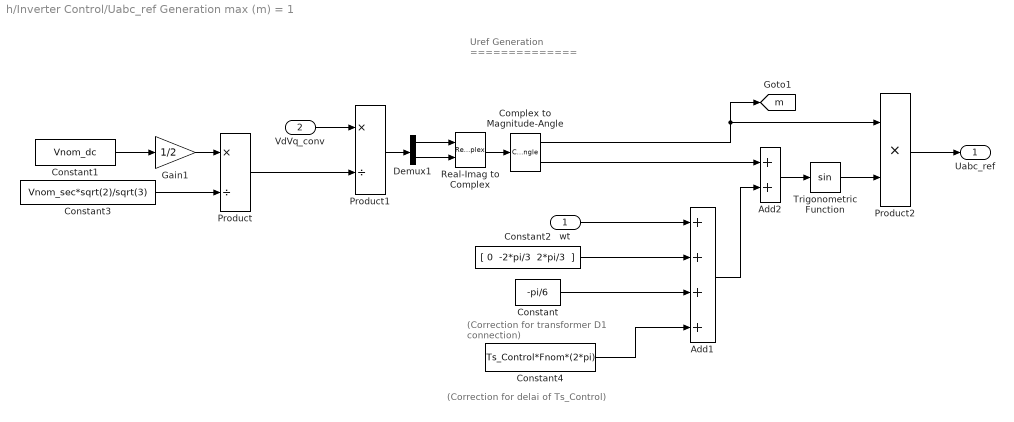
== system h/Inverter Control/Uabc_ref Generation max (m) = 1 ==
  note: (Correction for transformer
      |  D1 connection)
  note: (Correction for delai of Ts_Control)
  note: Uref Generation
      | ==============
  wt : Inport
  VdVq_conv : Inport  Port=2
  Add1 : Sum  Inputs=++++
  Add2 : Sum
  Complex to Magnitude-Angle : ComplexToMagnitudeAngle
  Constant : Constant  Value=-pi/6
  Constant1 : Constant  Value=Vnom_dc
  Constant2 : Constant  Value="[ 0  -2*pi/3  2*pi/3  ]"
  Constant3 : Constant  Value=Vnom_sec*sqrt(2)/sqrt(3)
  Constant4 : Constant  Value=Ts_Control*Fnom*(2*pi)
  Demux1 : Demux  Outputs=2
  Gain1 : Gain  Gain=1/2
  Product : Product  Inputs=*/  RndMeth=Zero
  Product1 : Product  Inputs=*/  RndMeth=Zero
  Product2 : Product  Inputs=**  RndMeth=Zero
  Real-Imag to Complex : RealImagToComplex
  Trigonometric Function : Trigonometry
  Uabc_ref : Outport  VectorParamsAs1DForOutWhenUnconnected=off
  tag scope: m=global
  wires:
  Constant1/1 -> Gain1/1
  VdVq_conv/1 -> Product1/1
  Product1/1 -> Demux1/1
  Gain1/1 -> Product/1
  Real-Imag to Complex/1 -> Complex to Magnitude-Angle/1
  Demux1/1 -> Real-Imag to Complex/1
  Demux1/2 -> Real-Imag to Complex/2
  Constant2/1 -> Add1/2
  Constant/1 -> Add1/3
  Constant3/1 -> Product/2
  Product/1 -> Product1/2
  Complex to Magnitude-Angle/2 -> Add2/1
  Add1/1 -> Add2/2
  Add2/1 -> Trigonometric Function/1
  Complex to Magnitude-Angle/1 -> [m], Product2/1
  Trigonometric Function/1 -> Product2/2
  Product2/1 -> Uabc_ref/1
  wt/1 -> Add1/1
  Constant4/1 -> Add1/4

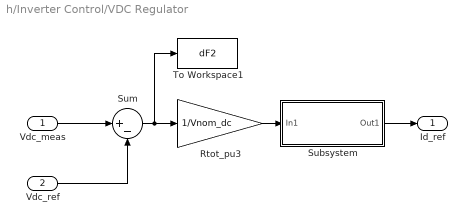
== system h/Inverter Control/VDC Regulator ==
  Vdc_meas : Inport  PortDimensions=1
  Vdc_ref : Inport  Port=2  PortDimensions=1
  Rtot_pu3 : Gain  Gain=1/Vnom_dc  SaturateOnIntegerOverflow=on  OutDataTypeStr=Inherit: Same as input  ParamDataTypeStr=Inherit: Same as input
  Subsystem : Subsystem
  Sum : Sum  Inputs=|+-
  To Workspace1 : ToWorkspace  VariableName=dF2  SampleTime=-1
  Id_ref : Outport  InitialOutput=0  VectorParamsAs1DForOutWhenUnconnected=off
  wires:
  Subsystem/1(Out1) -> Id_ref/1
  Rtot_pu3/1 -> Subsystem/1(In1)
  Vdc_ref/1 -> Sum/2
  Vdc_meas/1 -> Sum/1
  Sum/1 -> To Workspace1/1, Rtot_pu3/1

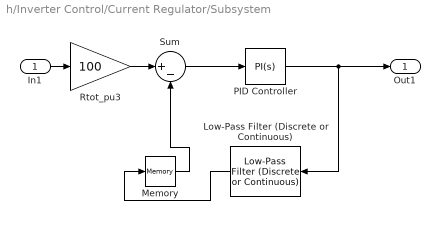
== system h/Inverter Control/Current Regulator/Subsystem ==
  In1 : Inport
  Low-Pass Filter (Discrete or Continuous) : eeGeneralControl/Low-Pass Filter (Discrete or Continuous)  K=30  T=1  B=inf  A=-inf  init_option=Inherited from block input  x0=0  Ts=-1
  Memory : Memory
  PID Controller : slpidlib/PID Controller  Controller=PI  Form=Parallel  TimeDomain=Continuous-time  UseExternalTs=off  SampleTime=-1  IntegratorMethod=Forward Euler  FilterMethod=Forward Euler  ControllerParametersSource=internal  P=0.000846  I=0.0103  UseKiTs=off  D=0  UseExternalDerivativeSource=off  N=100  UseFilter=on  TunerSelectOption=Transfer Function Based (PID Tuner App)  InitialConditionSource=internal  InitialConditionForIntegrator=0  InitialConditionForFilter=0  DifferentiatorICPrevScaledInput=0  ExternalReset=none  TrackingMode=off  Kt=1  LimitOutput=off  SatLimitsSource=internal  UpperSaturationLimit=inf  LowerSaturationLimit=-inf  LinearizeAsGain=on  AntiWindupMode=none  Kb=1  LimitIntegrator=off  UpperIntegratorSaturationLimit=inf  LowerIntegratorSaturationLimit=-inf  POutMin=[]  POutMax=[]  IOutMin=[]  IOutMax=[]  DOutMin=[]  DOutMax=[]  NOutMin=[]  NOutMax=[]  SumOutMin=[]  SumOutMax=[]  SaturationOutMin=[]  SaturationOutMax=[]  PParamMin=[]  PParamMax=[]  IParamMin=[]  IParamMax=[]  DParamMin=[]  DParamMax=[]  NParamMin=[]  NParamMax=[]  KbParamMin=[]  KbParamMax=[]  KtParamMin=[]  KtParamMax=[]  KbOutMin=[]  KbOutMax=[]  KtOutMin=[]  KtOutMax=[]  IntegratorOutMin=[]  IntegratorOutMax=[]  FilterOutMin=[]  FilterOutMax=[]  SumI1OutMin=[]  SumI1OutMax=[]  SumI2OutMin=[]  SumI2OutMax=[]  SumI3OutMin=[]  SumI3OutMax=[]  SumI4OutMin=[]  SumI4OutMax=[]  SumDOutMin=[]  SumDOutMax=[]  DifferentiatorOutMin=[]  DifferentiatorOutMax=[]  FilterDiffOutCoefMin=[]  FilterDiffOutCoefMax=[]  ReciprocalOutMin=[]  ReciprocalOutMax=[]  SumDenOutMin=[]  SumDenOutMax=[]  SumNumOutMin=[]  SumNumOutMax=[]  DivideOutMin=[]  DivideOutMax=[]  UdiffTsProdOutMin=[]  UdiffTsProdOutMax=[]  NTsProdOutMin=[]  NTsProdOutMax=[]  UintegralTsProdOutMin=[]  UintegralTsProdOutMax=[]  UngainTsProdOutMin=[]  UngainTsProdOutMax=[]  ClampingZeroOutDataTypeStr=Inherit: Inherit via back propagation  ClampingZeroOutMin=[]  ClampingZeroOutMax=[]  FilterDenConstantOutDataTypeStr=Inherit: Inherit via back propagation  FilterDenConstantOutMin=[]  FilterDenConstantOutMax=[]  PCopyOutDataTypeStr=Inherit: Inherit via back propagation  PCopyOutMin=[]  PCopyOutMax=[]  NCopyOutDataTypeStr=Inherit: Inherit via back propagation  NCopyOutMin=[]  NCopyOutMax=[]  IntegratorContinuousStateAttributes=''  IntegratorStateMustResolveToSignalObject=off  IntegratorRTWStateStorageClass=Auto  FilterContinuousStateAttributes=''  FilterStateMustResolveToSignalObject=off  FilterRTWStateStorageClass=Auto  ParallelPVariant=InternalParameters  IdealPVariant=Disabled  IVariant=InternalParameters  DVariant=Disabled  IntegratorVariant=Continuous  SatVariant=Disabled  AWVariant=Passthrough  PCopyVariant=Disabled  TRVariant=Disabled  FdbkBlocksVariant=Forward  IdealPFdbkVariant=Disabled  SatFdbkVariant=Disabled  DerivativeFilterVariant=Disabled  NVariant=Disabled  NCopyVariant=Disabled_SignalSpec  FilterICVariant=Disabled  IntegratorICVariant=InternalICs  ExternalResetVariant=Disabled  TRSumVariant=Passthrough  SumFdbkVariant=Disabled  SumVariant=Sum_PI  TsampFilterVariant=InternalTs  TsampNgainVariant=Passthrough  TsampIntegralVariant=Disabled_SignalSpec  ExternalSaturationOutDataTypeStr=Inherit: Same as second input  DerivativeSourceVariant=Disabled
  Rtot_pu3 : Gain  Gain=100  SaturateOnIntegerOverflow=on  OutDataTypeStr=Inherit: Same as input  ParamDataTypeStr=Inherit: Same as input
  Sum : Sum  Inputs=|+-
  Out1 : Outport  VectorParamsAs1DForOutWhenUnconnected=off
  wires:
  Sum/1 -> PID Controller/1
  PID Controller/1 -> Low-Pass Filter (Discrete or Continuous)/1, Out1/1
  In1/1 -> Rtot_pu3/1
  Rtot_pu3/1 -> Sum/1
  Memory/1 -> Sum/2
  Low-Pass Filter (Discrete or Continuous)/1 -> Memory/1

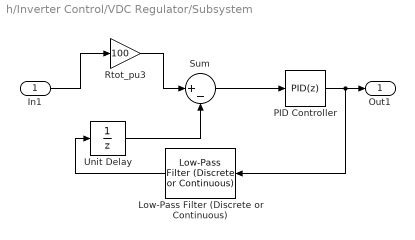
== system h/Inverter Control/VDC Regulator/Subsystem ==
  In1 : Inport
  Low-Pass Filter (Discrete or Continuous) : eeGeneralControl/Low-Pass Filter (Discrete or Continuous)  K=30  T=1  B=inf  A=-inf  init_option=Inherited from block input  x0=0  Ts=-1
  PID Controller : slpidlib/PID Controller  Controller=PID  Form=Parallel  TimeDomain=Discrete-time  UseExternalTs=off  SampleTime=-1  IntegratorMethod=Forward Euler  FilterMethod=Forward Euler  ControllerParametersSource=internal  P=k1  I=k2  UseKiTs=off  D=0  UseExternalDerivativeSource=off  N=100  UseFilter=on  TunerSelectOption=Transfer Function Based (PID Tuner App)  InitialConditionSource=internal  InitialConditionForIntegrator=0  InitialConditionForFilter=0  DifferentiatorICPrevScaledInput=0  ExternalReset=none  TrackingMode=off  Kt=1  LimitOutput=off  SatLimitsSource=internal  UpperSaturationLimit=inf  LowerSaturationLimit=-inf  LinearizeAsGain=on  AntiWindupMode=none  Kb=1  LimitIntegrator=off  UpperIntegratorSaturationLimit=inf  LowerIntegratorSaturationLimit=-inf  POutMin=[]  POutMax=[]  IOutMin=[]  IOutMax=[]  DOutMin=[]  DOutMax=[]  NOutMin=[]  NOutMax=[]  SumOutMin=[]  SumOutMax=[]  SaturationOutMin=[]  SaturationOutMax=[]  PParamMin=[]  PParamMax=[]  IParamMin=[]  IParamMax=[]  DParamMin=[]  DParamMax=[]  NParamMin=[]  NParamMax=[]  KbParamMin=[]  KbParamMax=[]  KtParamMin=[]  KtParamMax=[]  KbOutMin=[]  KbOutMax=[]  KtOutMin=[]  KtOutMax=[]  IntegratorOutMin=[]  IntegratorOutMax=[]  FilterOutMin=[]  FilterOutMax=[]  SumI1OutMin=[]  SumI1OutMax=[]  SumI2OutMin=[]  SumI2OutMax=[]  SumI3OutMin=[]  SumI3OutMax=[]  SumI4OutMin=[]  SumI4OutMax=[]  SumDOutMin=[]  SumDOutMax=[]  DifferentiatorOutMin=[]  DifferentiatorOutMax=[]  FilterDiffOutCoefMin=[]  FilterDiffOutCoefMax=[]  ReciprocalOutMin=[]  ReciprocalOutMax=[]  SumDenOutMin=[]  SumDenOutMax=[]  SumNumOutMin=[]  SumNumOutMax=[]  DivideOutMin=[]  DivideOutMax=[]  UdiffTsProdOutMin=[]  UdiffTsProdOutMax=[]  NTsProdOutMin=[]  NTsProdOutMax=[]  UintegralTsProdOutMin=[]  UintegralTsProdOutMax=[]  UngainTsProdOutMin=[]  UngainTsProdOutMax=[]  ClampingZeroOutDataTypeStr=Inherit: Inherit via back propagation  ClampingZeroOutMin=[]  ClampingZeroOutMax=[]  FilterDenConstantOutDataTypeStr=Inherit: Inherit via back propagation  FilterDenConstantOutMin=[]  FilterDenConstantOutMax=[]  PCopyOutDataTypeStr=Inherit: Inherit via back propagation  PCopyOutMin=[]  PCopyOutMax=[]  NCopyOutDataTypeStr=Inherit: Inherit via back propagation  NCopyOutMin=[]  NCopyOutMax=[]  IntegratorContinuousStateAttributes=''  IntegratorStateMustResolveToSignalObject=off  IntegratorRTWStateStorageClass=Auto  FilterContinuousStateAttributes=''  FilterStateMustResolveToSignalObject=off  FilterRTWStateStorageClass=Auto  ParallelPVariant=InternalParameters  IdealPVariant=Disabled  IVariant=InternalParameters  DVariant=InternalParameters  IntegratorVariant=Discrete  SatVariant=Disabled  AWVariant=Passthrough  PCopyVariant=Disabled  TRVariant=Disabled  FdbkBlocksVariant=Forward  IdealPFdbkVariant=Disabled  SatFdbkVariant=Disabled  DerivativeFilterVariant=ForwardEulerFilter  NVariant=InternalParameters  NCopyVariant=Disabled  FilterICVariant=InternalICsFilter  IntegratorICVariant=InternalICs  ExternalResetVariant=Disabled  TRSumVariant=Passthrough  SumFdbkVariant=Disabled  SumVariant=Sum_PID  TsampFilterVariant=InternalTs  TsampNgainVariant=Passthrough  TsampIntegralVariant=Disabled_SignalSpec  ExternalSaturationOutDataTypeStr=Inherit: Same as second input  DerivativeSourceVariant=ErrorSignal
  Rtot_pu3 : Gain  Gain=100  SaturateOnIntegerOverflow=on  OutDataTypeStr=Inherit: Same as input  ParamDataTypeStr=Inherit: Same as input
  Sum : Sum  Inputs=|+-
  Unit Delay : UnitDelay  InitialCondition=1  SampleTime=-1  HasFrameUpgradeWarning=on
  Out1 : Outport  VectorParamsAs1DForOutWhenUnconnected=off
  wires:
  PID Controller/1 -> Low-Pass Filter (Discrete or Continuous)/1, Out1/1
  Sum/1 -> PID Controller/1
  Low-Pass Filter (Discrete or Continuous)/1 -> Unit Delay/1
  Rtot_pu3/1 -> Sum/1
  In1/1 -> Rtot_pu3/1
  Unit Delay/1 -> Sum/2

== matlab function h/Inverter Control/MPPT Controller using Perturbe & Observe technique  ==
  settings: updateMethod=DISCRETE  sampleTime=Ts_Control
  data: Param input; Enabled input; V input; I input; D output
function D  = PandO(Param, Enabled, V, I)

% MPPT controller based on the Perturb & Observe algorithm.

% D output = Reference for DC link voltage (Vdc_ref) 
%
% Enabled input = 1 to enable the MPPT controller
% V input = PV array terminal voltage (V)
% I input = PV array current (A)
%
% Param input:
Dinit = Param(1);  %Initial value for Vdc_ref
Dmax = Param(2);   %Maximum value for Vdc_ref
Dmin = Param(3);   %Minimum value for Vdc_ref
deltaD = Param(4); %Increment value used to increase/decrease Vdc_ref
%  

persistent Vold Pold Dold;

dataType = 'double';

if isempty(Vold)
    Vold=0;
    Pold=0;
    Dold=Dinit;
end
P= V*I;
dV= V - Vold;
dP= P - Pold;

if dP ~= 0 & Enabled ~=0
    if dP < 0
        if dV < 0
            D = Dold + deltaD;
        else
            D = Dold - deltaD;
        end
    else
        if dV < 0
            D = Dold - deltaD;
        else
            D = Dold + deltaD;
        end    
    end
else D=Dold;
end

if D >= Dmax | D<= Dmin
    D=Dold;
end

Dold=D;
Vold=V;
Pold=P;
